simulink model "MVBMasterTransfer"  (R2014a)
settings: Solver=FixedStepDiscrete  StartTime=0.0  StopTime=100.0  FixedStep=1  RelTol=1e-3
settings Model: Creator=Administrator  LastModifiedBy=Administrator

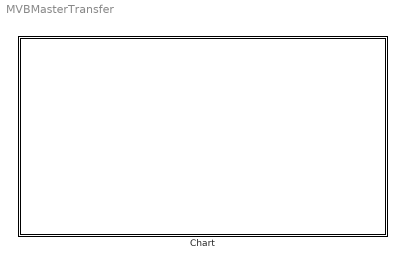
== system MVBMasterTransfer ==
  Chart : Stateflow chart  TreatAsAtomicUnit=on

== stateflow chart MVBMasterTransfer/Chart ==
  state MasterShip
    state OneMVB1 [parallel]
      settings: executionOrder=1
      state Timer [parallel]
        settings: executionOrder=2
        state BController [parallel]
          settings: executionOrder=1
          state AC [parallel]
            settings: executionOrder=1
            state T_standby_timer
            (default) -> MasterShip.OneMVB1.Timer.BController.AC.T_standby_timer
            MasterShip.OneMVB1.Timer.BController.AC.T_standby_timer -> MasterShip.OneMVB1.Timer.BController.AC.T_standby_timer [order 2] : stop_standby_timer/{run=0;}
            MasterShip.OneMVB1.Timer.BController.AC.T_standby_timer -> MasterShip.OneMVB1.Timer.BController.AC.T_standby_timer [order 1] : start_standby_timer/{run=1;}
            MasterShip.OneMVB1.Timer.BController.AC.T_standby_timer -> MasterShip.OneMVB1.Timer.BController.AC.T_standby_timer [order 3] : [run==1 && after(5,sec)]/{T_standby_event;}
          state BC [parallel]
            settings: executionOrder=2
            state T_master_turn_timer
            (default) -> MasterShip.OneMVB1.Timer.BController.BC.T_master_turn_timer
            MasterShip.OneMVB1.Timer.BController.BC.T_master_turn_timer -> MasterShip.OneMVB1.Timer.BController.BC.T_master_turn_timer [order 2] : stop_master_turn/{run=0;}
            MasterShip.OneMVB1.Timer.BController.BC.T_master_turn_timer -> MasterShip.OneMVB1.Timer.BController.BC.T_master_turn_timer [order 1] : start_master_turn/{run=1;}
            MasterShip.OneMVB1.Timer.BController.BC.T_master_turn_timer -> MasterShip.OneMVB1.Timer.BController.BC.T_master_turn_timer [order 3] : [run==1 && after(5,sec)]/{master_turn_over_event;}
          state CC [parallel]
            settings: executionOrder=3
            state resign_event_watcher
            (default) -> MasterShip.OneMVB1.Timer.BController.CC.resign_event_watcher
            MasterShip.OneMVB1.Timer.BController.CC.resign_event_watcher -> MasterShip.OneMVB1.Timer.BController.CC.resign_event_watcher [order 1] : trigger_freq_event[resign==0]/{canpatch = 1;}
            MasterShip.OneMVB1.Timer.BController.CC.resign_event_watcher -> MasterShip.OneMVB1.Timer.BController.CC.resign_event_watcher [order 2] : [resign==1 && canpatch == 1]/{resign_event;canpatch=0;}
        state AController [parallel]
          settings: executionOrder=2
          state DC [parallel]
            settings: executionOrder=1
            state T_interim_timer
            (default) -> MasterShip.OneMVB1.Timer.AController.DC.T_interim_timer
            MasterShip.OneMVB1.Timer.AController.DC.T_interim_timer -> MasterShip.OneMVB1.Timer.AController.DC.T_interim_timer [order 2] : stop_interim_timer/{run=0;}
            MasterShip.OneMVB1.Timer.AController.DC.T_interim_timer -> MasterShip.OneMVB1.Timer.AController.DC.T_interim_timer [order 1] : start_interim_timer/{run=1;}
            MasterShip.OneMVB1.Timer.AController.DC.T_interim_timer -> MasterShip.OneMVB1.Timer.AController.DC.T_interim_timer [order 3] : [run==1 && after(3,sec)]/{T_interim_event;}
          state EC [parallel]
            settings: executionOrder=2
            state T_find_timer
            (default) -> MasterShip.OneMVB1.Timer.AController.EC.T_find_timer
            MasterShip.OneMVB1.Timer.AController.EC.T_find_timer -> MasterShip.OneMVB1.Timer.AController.EC.T_find_timer [order 2] : stop_find_timer/{run=0;}
            MasterShip.OneMVB1.Timer.AController.EC.T_find_timer -> MasterShip.OneMVB1.Timer.AController.EC.T_find_timer [order 1] : start_find_timer/{run=1;}
            MasterShip.OneMVB1.Timer.AController.EC.T_find_timer -> MasterShip.OneMVB1.Timer.AController.EC.T_find_timer [order 3] : [run==1 && after(5,sec)]/{T_find_next;}
          state UltimateController [parallel]
            settings: executionOrder=3
            state The_Time
            (default) -> MasterShip.OneMVB1.Timer.AController.UltimateController.The_Time
            MasterShip.OneMVB1.Timer.AController.UltimateController.The_Time -> MasterShip.OneMVB1.Timer.AController.UltimateController.The_Time : [after(1,sec)]/{send(trigger_freq_event,OneMVB1.Timer.BController.CC);}
      state Chnannel [parallel]
        settings: executionOrder=3
        state Master_Frame
        MasterShip.OneMVB1.Chnannel.Master_Frame -> MasterShip.OneMVB1.Chnannel.Master_Frame [order 2] : Master_Frame_Input[master_frame_error==1]/{valid_master_frame=0;send(master_frame_event,OneMVB1.LOGIC);}
        (default) -> MasterShip.OneMVB1.Chnannel.Master_Frame
        MasterShip.OneMVB1.Chnannel.Master_Frame -> MasterShip.OneMVB1.Chnannel.Master_Frame [order 3] : Master_Frame_Input[master_frame_error==0]/{valid_master_frame=valid_master_input;send(master_frame_event,OneMVB1.LOGIC);}
        MasterShip.OneMVB1.Chnannel.Master_Frame -> MasterShip.OneMVB1.Chnannel.Master_Frame [order 1] : Master_Frame_Input[master_frame_error==2]
      state LOGIC [parallel]
        settings: executionOrder=1
        state initial
        state Standby_Master
          entry:send(start_standby_timer,Timer);
          exit:send(stop_standby_timer,Timer);
        state Rrgular_Master
          entry:send(start_master_turn,Timer);
          exit:send(stop_master_turn,Timer);
        state st
        state bt
        state sr
        state Interim_Master
          entry:send(start_interim_timer,Timer);
          exit:send(stop_interim_timer,Timer);
        state Find_Next
          entry:send(start_find_timer,Timer);
          exit:send(stop_find_timer,Timer);
        state T_F
        (default) -> initial
        MasterShip.OneMVB1.LOGIC.Rrgular_Master -> MasterShip.OneMVB1.LOGIC.Standby_Master [order 1] : master_frame_event[ReqId == CNMasterShip || ReqId == CNStatusRequest]/{HasMasterFrame=1;}
        initial -> MasterShip.OneMVB1.LOGIC.Standby_Master
        MasterShip.OneMVB1.LOGIC.Standby_Master -> MasterShip.OneMVB1.LOGIC.Rrgular_Master [order 3] : T_standby_event
        MasterShip.OneMVB1.LOGIC.Rrgular_Master -> MasterShip.OneMVB1.LOGIC.Standby_Master [order 2] : resign_event
        MasterShip.OneMVB1.LOGIC.st -> MasterShip.OneMVB1.LOGIC.Standby_Master : /{status_response_type=1;status_response_event;}
        (junction 520) -> MasterShip.OneMVB1.LOGIC.Standby_Master
        (junction 519) -> MasterShip.OneMVB1.LOGIC.Standby_Master
        (junction 514) -> MasterShip.OneMVB1.LOGIC.Standby_Master [order 2]
        (junction 518) -> MasterShip.OneMVB1.LOGIC.Standby_Master [order 3] : /{status_response_type=2}
        MasterShip.OneMVB1.LOGIC.Standby_Master -> (junction 514) [order 1] : master_frame_event[valid_master_frame == 1]
        MasterShip.OneMVB1.LOGIC.Standby_Master -> (junction 514) [order 2] : [HasMasterFrame==1 && valid_master_frame == 1]/{HasMasterFrame=0;}
        (junction 515) -> MasterShip.OneMVB1.LOGIC.Standby_Master [order 2]
        MasterShip.OneMVB1.LOGIC.bt -> MasterShip.OneMVB1.LOGIC.Rrgular_Master : /{CurrentMasterId=CNMVBId;bemaster_response_event;}
        (junction 516) -> MasterShip.OneMVB1.LOGIC.Rrgular_Master [order 1] : [BAitr>BAlen]/{BAitr=0;}
        MasterShip.OneMVB1.LOGIC.Rrgular_Master -> (junction 517) [order 3] : master_turn_over_event
        (junction 518) -> MasterShip.OneMVB1.LOGIC.st [order 2] : [ReqId == CNStatusRequest]
        (junction 515) -> MasterShip.OneMVB1.LOGIC.bt [order 1] : [CNACT == 1]
        (junction 514) -> (junction 518) [order 1] : [RevMVBId == CNMVBId]
        (junction 518) -> (junction 515) [order 1] : [ReqId == CNMasterShip]
        (junction 517) -> (junction 516) [order 2] : /{BAitr=BAitr+1;}
        (junction 517) -> (junction 516) [order 1] : [BAitr==CNMVBId-1]/{BAitr=BAitr+2;}
        (junction 516) -> MasterShip.OneMVB1.LOGIC.Find_Next [order 2] : /{ReqId=CNStatusRequest;RevMVBId = BAitr;Master_Frame_Input;}
        MasterShip.OneMVB1.LOGIC.T_F -> (junction 517)
        MasterShip.OneMVB1.LOGIC.Find_Next -> MasterShip.OneMVB1.LOGIC.sr [order 1] : status_response_event[status_response_type == 1]
        MasterShip.OneMVB1.LOGIC.sr -> MasterShip.OneMVB1.LOGIC.Interim_Master : /{ReqId=CNMasterShip;RevMVBId=BAitr;Master_Frame_Input;}
        MasterShip.OneMVB1.LOGIC.Interim_Master -> (junction 519) [order 2] : T_interim_event/{error = 1;}
        MasterShip.OneMVB1.LOGIC.Interim_Master -> (junction 520) [order 1] : bemaster_response_event[CurrentMasterId != CNMVBId]/{error = 0;}
        MasterShip.OneMVB1.LOGIC.Find_Next -> MasterShip.OneMVB1.LOGIC.T_F [order 3] : status_response_event[status_response_type>=2]
        MasterShip.OneMVB1.LOGIC.Interim_Master -> (junction 520) [order 3] : bemaster_response_event[CurrentMasterId == CNMVBId]/{error = 1;}
        MasterShip.OneMVB1.LOGIC.Find_Next -> MasterShip.OneMVB1.LOGIC.T_F [order 2] : T_find_next
    state OneMVB2 [parallel]
      settings: executionOrder=2
      state Chnannel [parallel]
        settings: executionOrder=3
        state Master_Frame
        MasterShip.OneMVB2.Chnannel.Master_Frame -> MasterShip.OneMVB2.Chnannel.Master_Frame [order 2] : Master_Frame_Input[master_frame_error==1]/{valid_master_frame=0;send(master_frame_event,OneMVB2.LOGIC);}
        (default) -> MasterShip.OneMVB2.Chnannel.Master_Frame
        MasterShip.OneMVB2.Chnannel.Master_Frame -> MasterShip.OneMVB2.Chnannel.Master_Frame [order 3] : Master_Frame_Input[master_frame_error==0]/{valid_master_frame=valid_master_input;send(master_frame_event,OneMVB2.LOGIC);}
        MasterShip.OneMVB2.Chnannel.Master_Frame -> MasterShip.OneMVB2.Chnannel.Master_Frame [order 1] : Master_Frame_Input[master_frame_error==2]
      state Timer [parallel]
        settings: executionOrder=2
        state BController [parallel]
          settings: executionOrder=1
          state AC [parallel]
            settings: executionOrder=1
            state T_standby_timer
            (default) -> MasterShip.OneMVB2.Timer.BController.AC.T_standby_timer
            MasterShip.OneMVB2.Timer.BController.AC.T_standby_timer -> MasterShip.OneMVB2.Timer.BController.AC.T_standby_timer [order 2] : stop_standby_timer/{run=0;}
            MasterShip.OneMVB2.Timer.BController.AC.T_standby_timer -> MasterShip.OneMVB2.Timer.BController.AC.T_standby_timer [order 1] : start_standby_timer/{run=1;}
            MasterShip.OneMVB2.Timer.BController.AC.T_standby_timer -> MasterShip.OneMVB2.Timer.BController.AC.T_standby_timer [order 3] : [run==1 && after(11,sec)]/{T_standby_event;}
          state BC [parallel]
            settings: executionOrder=2
            state T_master_turn_timer
            (default) -> MasterShip.OneMVB2.Timer.BController.BC.T_master_turn_timer
            MasterShip.OneMVB2.Timer.BController.BC.T_master_turn_timer -> MasterShip.OneMVB2.Timer.BController.BC.T_master_turn_timer [order 2] : stop_master_turn/{run=0;}
            MasterShip.OneMVB2.Timer.BController.BC.T_master_turn_timer -> MasterShip.OneMVB2.Timer.BController.BC.T_master_turn_timer [order 1] : start_master_turn/{run=1;}
            MasterShip.OneMVB2.Timer.BController.BC.T_master_turn_timer -> MasterShip.OneMVB2.Timer.BController.BC.T_master_turn_timer [order 3] : [run==1 && after(4,sec)]/{master_turn_over_event;}
          state CC [parallel]
            settings: executionOrder=3
            state resign_event_watcher
            (default) -> MasterShip.OneMVB2.Timer.BController.CC.resign_event_watcher
            MasterShip.OneMVB2.Timer.BController.CC.resign_event_watcher -> MasterShip.OneMVB2.Timer.BController.CC.resign_event_watcher [order 1] : trigger_freq_event[resign==0]/{canpatch = 1;}
            MasterShip.OneMVB2.Timer.BController.CC.resign_event_watcher -> MasterShip.OneMVB2.Timer.BController.CC.resign_event_watcher [order 2] : [resign==1 && canpatch == 1]/{resign_event;canpatch=0;}
        state AController [parallel]
          settings: executionOrder=2
          state DC [parallel]
            settings: executionOrder=1
            state T_interim_timer
            (default) -> MasterShip.OneMVB2.Timer.AController.DC.T_interim_timer
            MasterShip.OneMVB2.Timer.AController.DC.T_interim_timer -> MasterShip.OneMVB2.Timer.AController.DC.T_interim_timer [order 2] : stop_interim_timer/{run=0;}
            MasterShip.OneMVB2.Timer.AController.DC.T_interim_timer -> MasterShip.OneMVB2.Timer.AController.DC.T_interim_timer [order 1] : start_interim_timer/{run=1;}
            MasterShip.OneMVB2.Timer.AController.DC.T_interim_timer -> MasterShip.OneMVB2.Timer.AController.DC.T_interim_timer [order 3] : [run==1 && after(5,sec)]/{T_interim_event;}
          state EC [parallel]
            settings: executionOrder=2
            state T_find_timer
            (default) -> MasterShip.OneMVB2.Timer.AController.EC.T_find_timer
            MasterShip.OneMVB2.Timer.AController.EC.T_find_timer -> MasterShip.OneMVB2.Timer.AController.EC.T_find_timer [order 2] : stop_find_timer/{run=0;}
            MasterShip.OneMVB2.Timer.AController.EC.T_find_timer -> MasterShip.OneMVB2.Timer.AController.EC.T_find_timer [order 1] : start_find_timer/{run=1;}
            MasterShip.OneMVB2.Timer.AController.EC.T_find_timer -> MasterShip.OneMVB2.Timer.AController.EC.T_find_timer [order 3] : [run==1 && after(5,sec)]/{T_find_next;}
          state UltimateController [parallel]
            settings: executionOrder=3
            state The_Time
            (default) -> MasterShip.OneMVB2.Timer.AController.UltimateController.The_Time
            MasterShip.OneMVB2.Timer.AController.UltimateController.The_Time -> MasterShip.OneMVB2.Timer.AController.UltimateController.The_Time : [after(1,sec)]/{send(trigger_freq_event,OneMVB2.Timer.BController.CC);}
      state LOGIC [parallel]
        settings: executionOrder=1
        state ps
        state Standby_Master
          entry:send(start_standby_timer,Timer);
          exit:send(stop_standby_timer,Timer);
        state Rrgular_Master
          entry:send(start_master_turn,Timer);
          exit:send(stop_master_turn,Timer);
        state st
        state bt
        state sr
        state Interim_Master
          entry:send(start_interim_timer,Timer);
          exit:send(stop_interim_timer,Timer);
        state Find_Next
          entry:send(start_find_timer,Timer);
          exit:send(stop_find_timer,Timer);
        state T_F
        (default) -> ps
        MasterShip.OneMVB2.LOGIC.Rrgular_Master -> MasterShip.OneMVB2.LOGIC.Standby_Master [order 1] : master_frame_event[ReqId == CNMasterShip || ReqId == CNStatusRequest]/{HasMasterFrame=1;}
        MasterShip.OneMVB2.LOGIC.Standby_Master -> MasterShip.OneMVB2.LOGIC.Rrgular_Master [order 3] : T_standby_event
        ps -> MasterShip.OneMVB2.LOGIC.Standby_Master
        MasterShip.OneMVB2.LOGIC.Rrgular_Master -> MasterShip.OneMVB2.LOGIC.Standby_Master [order 2] : resign_event
        (junction 940) -> MasterShip.OneMVB2.LOGIC.Standby_Master [order 2]
        MasterShip.OneMVB2.LOGIC.st -> MasterShip.OneMVB2.LOGIC.Standby_Master : /{status_response_type=1;status_response_event;}
        (junction 945) -> MasterShip.OneMVB2.LOGIC.Standby_Master
        (junction 944) -> MasterShip.OneMVB2.LOGIC.Standby_Master
        (junction 939) -> MasterShip.OneMVB2.LOGIC.Standby_Master [order 2]
        (junction 943) -> MasterShip.OneMVB2.LOGIC.Standby_Master [order 3] : /{status_response_type=2}
        MasterShip.OneMVB2.LOGIC.Standby_Master -> (junction 939) [order 1] : master_frame_event[valid_master_frame == 1]
        MasterShip.OneMVB2.LOGIC.Standby_Master -> (junction 939) [order 2] : [HasMasterFrame==1 && valid_master_frame == 1]/{HasMasterFrame=0;}
        MasterShip.OneMVB2.LOGIC.bt -> MasterShip.OneMVB2.LOGIC.Rrgular_Master : /{CurrentMasterId=CNMVBId;bemaster_response_event;}
        (junction 941) -> MasterShip.OneMVB2.LOGIC.Rrgular_Master [order 1] : [BAitr>BAlen]/{BAitr=0;}
        MasterShip.OneMVB2.LOGIC.Rrgular_Master -> (junction 942) [order 3] : master_turn_over_event
        (junction 943) -> MasterShip.OneMVB2.LOGIC.st [order 2] : [ReqId == CNStatusRequest]
        (junction 940) -> MasterShip.OneMVB2.LOGIC.bt [order 1] : [CNACT == 1]
        (junction 939) -> (junction 943) [order 1] : [RevMVBId == CNMVBId]
        (junction 943) -> (junction 940) [order 1] : [ReqId == CNMasterShip]
        (junction 942) -> (junction 941) [order 2] : /{BAitr=BAitr+1;}
        (junction 942) -> (junction 941) [order 1] : [BAitr==CNMVBId-1]/{BAitr=BAitr+2;}
        MasterShip.OneMVB2.LOGIC.T_F -> (junction 942)
        (junction 941) -> MasterShip.OneMVB2.LOGIC.Find_Next [order 2] : /{ReqId=CNStatusRequest;RevMVBId = BAitr;Master_Frame_Input;}
        MasterShip.OneMVB2.LOGIC.sr -> MasterShip.OneMVB2.LOGIC.Interim_Master : /{ReqId=CNMasterShip;RevMVBId=BAitr;Master_Frame_Input;}
        MasterShip.OneMVB2.LOGIC.Find_Next -> MasterShip.OneMVB2.LOGIC.sr [order 1] : status_response_event[status_response_type == 1]
        MasterShip.OneMVB2.LOGIC.Interim_Master -> (junction 944) [order 2] : T_interim_event/{error = 1;}
        MasterShip.OneMVB2.LOGIC.Interim_Master -> (junction 945) [order 1] : bemaster_response_event[CurrentMasterId != CNMVBId]/{error = 0;}
        MasterShip.OneMVB2.LOGIC.Find_Next -> MasterShip.OneMVB2.LOGIC.T_F [order 3] : status_response_event[status_response_type>=2]
        MasterShip.OneMVB2.LOGIC.Find_Next -> MasterShip.OneMVB2.LOGIC.T_F [order 2] : T_find_next
        MasterShip.OneMVB2.LOGIC.Interim_Master -> (junction 945) [order 3] : bemaster_response_event[CurrentMasterId == CNMVBId]/{error = 1;}
  (default) -> MasterShip
  data: turn local int32 =0; run local int32 =0; turn local int32 =0; run local int32 =0; canpatch local int32 =0; run local int32 =0; run local int32 =0; HasMasterFrame local int32 =0; CNMVBId local int32 =1; CNACT local int32 =1; turn local int32 =0; run local int32 =0; turn local int32 =0; run local int32 =0; canpatch local int32 =0; turn local int32 =0; run local int32 =0; turn local int32 =0; run local int32 =0; HasMasterFrame local int32 =0; CNMVBId local int32 =2; CNACT local int32 =1; run local int32 =0; RevMVBId local int32 =0; ReqId local int32 =0; status_response_type local int32 =0; T_alive local int32 =2; BAitr local int32 =0; BAlen local int32 =2; valid_master_input local int32 =1; CurrentMasterId local int32 =1; error local int32 =0; CNMasterShip local int32 =1; CNStatusRequest local int32 =2; T_RMTurn local int32 =8; resign local int32 =0; master_frame_error local int32 =0; valid_master_frame local int32 =1
  events: resign_watch_event local FUNCTION_CALL_EVENT; start_standby_timer local EITHER_EDGE_EVENT; stop_standby_timer local EITHER_EDGE_EVENT; start_master_turn local FUNCTION_CALL_EVENT; stop_master_turn local FUNCTION_CALL_EVENT; master_turn_over_event local FUNCTION_CALL_EVENT; T_standby_event local EITHER_EDGE_EVENT; T_find_next local EITHER_EDGE_EVENT; T_interim_event local EITHER_EDGE_EVENT; resign_event local FUNCTION_CALL_EVENT; start_interim_timer local FUNCTION_CALL_EVENT; stop_interim_timer local FUNCTION_CALL_EVENT; start_find_timer local FUNCTION_CALL_EVENT; stop_find_timer local FUNCTION_CALL_EVENT; master_frame_event local EITHER_EDGE_EVENT; trigger_freq_event local FUNCTION_CALL_EVENT; resign_watch_event local FUNCTION_CALL_EVENT; start_standby_timer local EITHER_EDGE_EVENT; stop_standby_timer local EITHER_EDGE_EVENT; start_master_turn local FUNCTION_CALL_EVENT; stop_master_turn local FUNCTION_CALL_EVENT; master_turn_over_event local FUNCTION_CALL_EVENT; T_standby_event local EITHER_EDGE_EVENT; T_find_next local EITHER_EDGE_EVENT; T_interim_event local EITHER_EDGE_EVENT; resign_event local FUNCTION_CALL_EVENT; start_interim_timer local FUNCTION_CALL_EVENT; stop_interim_timer local FUNCTION_CALL_EVENT; start_find_timer local FUNCTION_CALL_EVENT; stop_find_timer local FUNCTION_CALL_EVENT; master_frame_event local EITHER_EDGE_EVENT; trigger_freq_event local FUNCTION_CALL_EVENT; status_response_event local EITHER_EDGE_EVENT; bemaster_response_event local EITHER_EDGE_EVENT; Master_Frame_Input local FUNCTION_CALL_EVENT
